simulink model "ex2_qpsk_srrc_scope"  (R2017a)
settings: Solver=FixedStepAuto  StartTime=0  StopTime=100e-3  RelTol=1e-3
model workspace (MAT data in the model file):
  M = 4
  Rb = 1000
  beta = 0.3
  osf = 16
  span = 12
libraries: commfilt2 x2, commrandsrc3 x1, commdigbbndpm3 x1
settings Model: Creator=root  LastModifiedBy=root

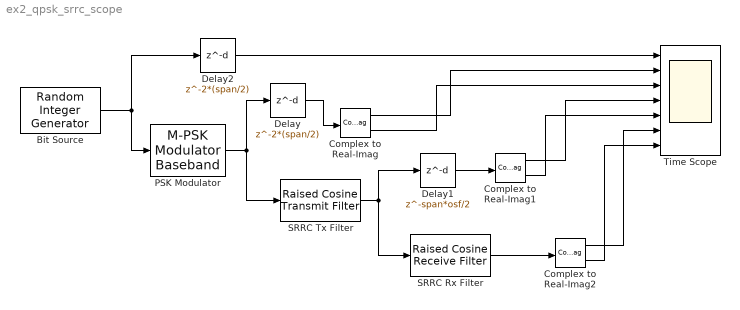
== system ex2_qpsk_srrc_scope ==
  Bit Source : commrandsrc3/Random Integer Generator  SetSize=2  SeedSource=Auto  Seed=1922  SampleTime=1/Rb  SamplesPerFrame=log2(M)  OutputDataType=uint8  SimulateUsing=Interpreted execution
  Complex to Real-Imag : ComplexToRealImag
  Complex to Real-Imag1 : ComplexToRealImag
  Complex to Real-Imag2 : ComplexToRealImag
  Delay : Delay  DelayLength=2*(span/2)  InitialCondition=0
  Delay1 : Delay  DelayLength=span*osf/2  InitialCondition=0
  Delay2 : Delay  DelayLength=2*(span/2)  InitialCondition=0
  PSK Modulator : commdigbbndpm3/M-PSK Modulator Baseband  M=M  InType=Bit  Enc=Gray  Mapping=[0:7]  Ph=pi/M  outDtype=double  outWordLen=16  outUDDataType=sfix(16)  outFracLenMode=Best precision  outFracLen=15  outDataTypeStr=double  outLastDataTypeStr=double
      settings: SourceProductName=Communications System Toolbox
  SRRC Rx Filter : commfilt2/Raised Cosine Receive Filter  filtType=Square root  R=beta  filtSpan=span  N=osf  downFactor=1  downOffset=0  filterGain=1  RateOptions=Allow multirate processing  framing=Mute  checkCoeff=off  variableName=rcRxFilt  currentFiltSpan=span  D=(span)/2  inputOffset=0  sampMode=Mute  saveAsFlag=0  rateMode=Downsampling  checkGain=Normalized  launchFVT=on  roundingMode=Floor  overflowMode=off  coeffDataTypeStr=Inherit: Same word length as input  coeffMin=[]  coeffMax=[]  coeffLastDataTypeStr=Inherit: Same word length as input  accumDataTypeStr=Inherit: Same as product output  accumLastDataTypeStr=Inherit: Same as product output  outputDataTypeStr=Inherit: Same as accumulator  outputMin=[]  outputMax=[]  outputLastDataTypeStr=Inherit: Same as accumulator
  SRRC Tx Filter : commfilt2/Raised Cosine Transmit Filter  filtType=Square root  R=beta  filtSpan=span  N=osf  filterGain=1  RateOptions=Allow multirate processing  framing=Mute  checkCoeff=off  variableName=rcTxFilt  checkGain=Normalized  sampMode=Mute  saveAsFlag=0  currentFiltSpan=span  D=(span)/2  launchFVT=on  roundingMode=Floor  overflowMode=off  coeffDataTypeStr=Inherit: Same word length as input  coeffMin=[]  coeffMax=[]  coeffLastDataTypeStr=Inherit: Same word length as input  outputDataTypeStr=Inherit: Same as accumulator  outputMin=[]  outputMax=[]  outputLastDataTypeStr=Inherit: Same as accumulator
  Time Scope : Scope  NumInputPorts=7
  wires:
  Bit Source/1 -> Delay2/1, PSK Modulator/1
  PSK Modulator/1 -> Delay/1, SRRC Tx Filter/1
  SRRC Tx Filter/1 -> Delay1/1, SRRC Rx Filter/1
  Complex to Real-Imag1/1 -> Time Scope/4
  Complex to Real-Imag1/2 -> Time Scope/5
  Delay/1 -> Complex to Real-Imag/1
  Complex to Real-Imag/1 -> Time Scope/2
  Complex to Real-Imag/2 -> Time Scope/3
  Delay1/1 -> Complex to Real-Imag1/1
  Complex to Real-Imag2/1 -> Time Scope/6
  Complex to Real-Imag2/2 -> Time Scope/7
  SRRC Rx Filter/1 -> Complex to Real-Imag2/1
  Delay2/1 -> Time Scope/1
